simulink model "Bicycle_model"  (R2024b)
settings: Solver=FixedStepAuto  StartTime=0.0  StopTime=40  FixedStep=0.01  RelTol=1e-3
values from neighbouring files (symbols this model uses):
  a = 1.10    (= 1.1)    [Bicycle_model_parameters_formula.m]
  A = 1.80    (= 1.8)    [Bicycle_model_parameters_formula.m]
  a1f = -1e-5    (= -1e-05)    [Bicycle_model_parameters_formula.m]
  a1r = -1e-5    (= -1e-05)    [Bicycle_model_parameters_formula.m]
  a2f = 0.95    [Bicycle_model_parameters_formula.m]
  a2r = 0.95    [Bicycle_model_parameters_formula.m]
  b = L-a    (= 1.7)    [Bicycle_model_parameters_formula.m]
  Bf = 0.0813    [Bicycle_model_parameters_formula.m]
  Br = 0.0925    [Bicycle_model_parameters_formula.m]
  Cf = 1.2947    [Bicycle_model_parameters_formula.m]
  Cr = 1.2617    [Bicycle_model_parameters_formula.m]
  cz = 0    [Bicycle_model_parameters_formula.m]
  Ef = -8.3966    [Bicycle_model_parameters_formula.m]
  Er = -8.7012    [Bicycle_model_parameters_formula.m]
  g = 9.81    [Bicycle_model_parameters_formula.m]
  I = 3500    [Bicycle_model_parameters_formula.m]
  L = 2.8    [Bicycle_model_parameters_formula.m]
  m = 1650    [Bicycle_model_parameters_formula.m]
  rho = 1.225    [Bicycle_model_parameters_formula.m]
  SR = 10    [Bicycle_model_parameters_formula.m]
libraries: aerolibconvert2 x5, simulink x1
settings Model: Creator=jayku  LastModifiedBy=jayku

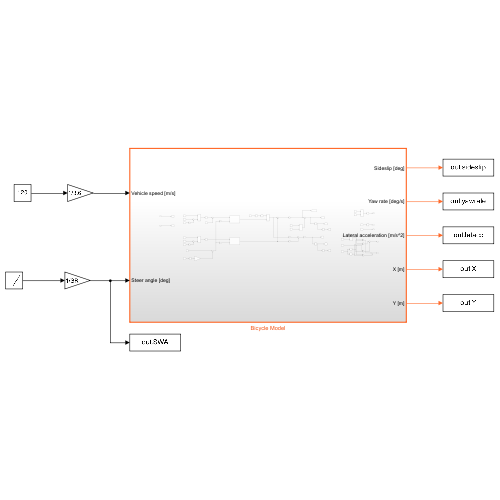
[thumbnail: Simulink's stored preview of the top-level diagram]
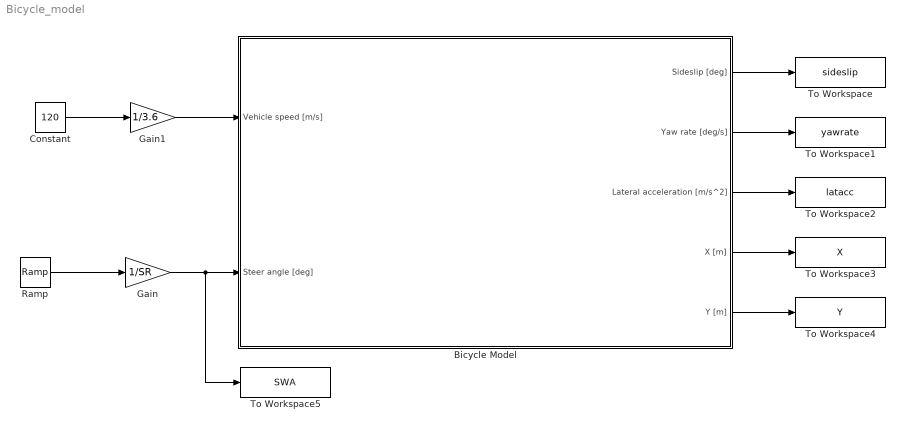
== system Bicycle_model ==
  Bicycle Model : Subsystem  TreatAsAtomicUnit=on
  Constant : Constant  Value=120
  Gain : Gain  Gain=1/SR
  Gain1 : Gain  Gain=1/3.6
  Ramp : simulink/Sources/Ramp  slope=2  start=0  InitialOutput=0
  To Workspace : ToWorkspace  VariableName=sideslip  SaveFormat=Timeseries  SampleTime=-1
  To Workspace1 : ToWorkspace  VariableName=yawrate  SaveFormat=Timeseries  SampleTime=-1
  To Workspace2 : ToWorkspace  VariableName=latacc  SaveFormat=Timeseries  SampleTime=-1
  To Workspace3 : ToWorkspace  VariableName=X  SaveFormat=Timeseries  SampleTime=-1
  To Workspace4 : ToWorkspace  VariableName=Y  SaveFormat=Timeseries  SampleTime=-1
  To Workspace5 : ToWorkspace  VariableName=SWA  SaveFormat=Timeseries  SampleTime=-1
  wires:
  Gain/1 -> To Workspace5/1, Bicycle Model/2(Steer angle [deg])
  Constant/1 -> Gain1/1
  Gain1/1 -> Bicycle Model/1(Vehicle speed [m/s])
  Ramp/1 -> Gain/1
  Bicycle Model/1(Sideslip [deg]) -> To Workspace/1
  Bicycle Model/2(Yaw rate [deg/s]) -> To Workspace1/1
  Bicycle Model/3(Lateral acceleration [m/s^2]) -> To Workspace2/1
  Bicycle Model/4(X [m]) -> To Workspace3/1
  Bicycle Model/5(Y [m]) -> To Workspace4/1

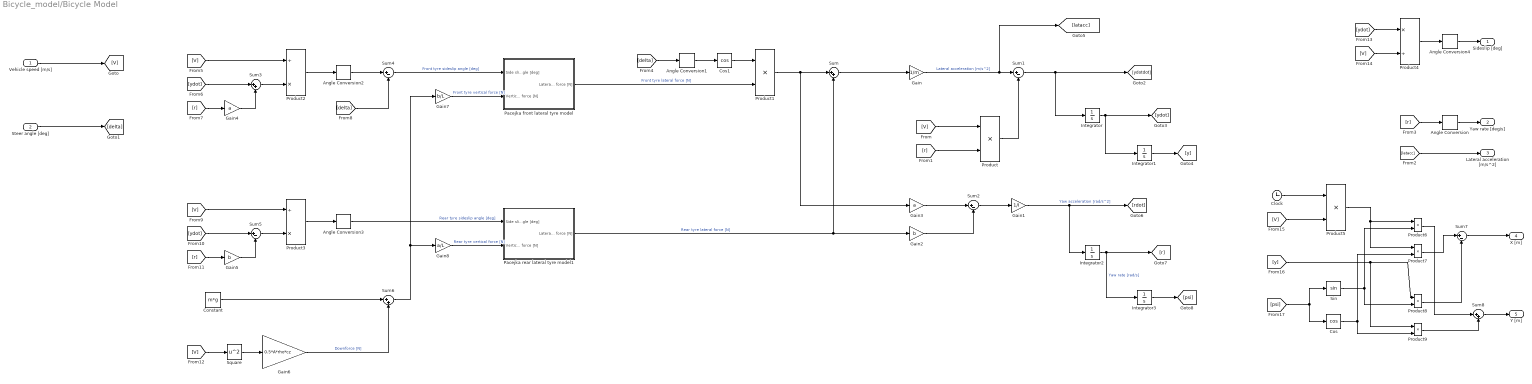
== system Bicycle_model/Bicycle Model ==
  Vehicle speed [m/s] : Inport
  Steer angle [deg] : Inport  Port=2
  Angle Conversion{,2..4} (4 alike) : aerolibconvert2/Angle Conversion  IU=rad  OU=deg
  Angle Conversion1 : aerolibconvert2/Angle Conversion  IU=deg  OU=rad
  Clock : Clock
  Constant : Constant  Value=m*g
  Cos : Trigonometry  Operator=cos
  Cos1 : Trigonometry  Operator=cos
  Gain : Gain  Gain=1/m
  Gain1 : Gain  Gain=1/I
  Gain2 : Gain  Gain=b
  Gain3 : Gain  Gain=a
  Gain4 : Gain  Gain=a
  Gain5 : Gain  Gain=b
  Gain6 : Gain  Gain=0.5*A*rho*cz
  Gain7 : Gain  Gain=b/L
  Gain8 : Gain  Gain=a/L
  Integrator{,1..3} (4 alike) : Integrator
  Pacejka front lateral tyre model : Subsystem
  Pacejka rear lateral tyre model1 : Subsystem
  Product{,1,5..9} (7 alike) : Product
  Product2 : Product  Inputs=/*
  Product3 : Product  Inputs=/*
  Product4 : Product  Inputs=*/
  Sin : Trigonometry
  Square : Math  Operator=square
  Sum{,3,6,8} (4 alike) : Sum  Inputs=|++
  Sum{1..2,4..5,7} (5 alike) : Sum  Inputs=|+-
  Sideslip [deg] : Outport
  Yaw rate [deg/s] : Outport  Port=2
  Lateral acceleration [m/s^2] : Outport  Port=3
  X [m] : Outport  Port=4
  Y [m] : Outport  Port=5
  wires:
  Vehicle speed [m/s]/1 -> [V]
  Sum/1 -> Gain/1
  Gain/1 -> [latacc], Sum1/1  "Lateral acceleration [m/s^2]"
  Product/1 -> Sum1/2
  [V] -> Product/1
  [r] -> Product/2
  Sum1/1 -> Integrator/1, [ydotdot]
  Integrator/1 -> Integrator1/1, [ydot]
  Integrator1/1 -> [y]
  [latacc] -> Lateral acceleration [m/s^2]/1
  Sum2/1 -> Gain1/1
  Gain1/1 -> Integrator2/1, [rdot]  "Yaw acceleration [rad/s^2]"
  Integrator2/1 -> [r], Integrator3/1  "Yaw rate [rad/s]"
  Integrator3/1 -> [psi]
  [r] -> Angle Conversion/1
  Angle Conversion/1 -> Yaw rate [deg/s]/1
  Gain3/1 -> Sum2/1
  Gain2/1 -> Sum2/2
  Pacejka rear lateral tyre model1/1(Lateral force [N]) -> Gain2/1, Sum/2  "Rear tyre lateral force [N]"
  Pacejka front lateral tyre model/1(Lateral force [N]) -> Product1/2  "Front tyre lateral force [N]"
  Product1/1 -> Gain3/1, Sum/1
  [delta] -> Angle Conversion1/1
  Cos1/1 -> Product1/1
  Angle Conversion1/1 -> Cos1/1
  [V] -> Product2/1
  [ydot] -> Sum3/1
  Sum3/1 -> Product2/2
  Gain4/1 -> Sum3/2
  [r] -> Gain4/1
  Product2/1 -> Angle Conversion2/1
  Angle Conversion2/1 -> Sum4/1
  [delta] -> Sum4/2
  Sum4/1 -> Pacejka front lateral tyre model/1(Side slip angle [deg])  "Front tyre sideslip angle [deg]"
  Sum5/1 -> Product3/2
  [V] -> Product3/1
  [r] -> Gain5/1
  [ydot] -> Sum5/1
  Product3/1 -> Angle Conversion3/1
  Gain5/1 -> Sum5/2
  Angle Conversion3/1 -> Pacejka rear lateral tyre model1/1(Side slip angle [deg])  "Rear tyre sideslip angle [deg]"
  Gain6/1 -> Sum6/2  "Downforce [N]"
  Constant/1 -> Sum6/1
  [V] -> Square/1
  Square/1 -> Gain6/1
  Gain8/1 -> Pacejka rear lateral tyre model1/2(Vertical force [N])  "Rear tyre vertical force [N]"
  Gain7/1 -> Pacejka front lateral tyre model/2(Vertical force [N])  "Front tyre vertical force [N]"
  Sum6/1 -> Gain7/1, Gain8/1
  Product4/1 -> Angle Conversion4/1
  Angle Conversion4/1 -> Sideslip [deg]/1
  [ydot] -> Product4/1
  [V] -> Product4/2
  Clock/1 -> Product5/1
  [V] -> Product5/2
  [psi] -> Sin/1, Cos/1
  Product5/1 -> Product7/1, Product6/1
  Sin/1 -> Product6/2, Product8/2
  Cos/1 -> Product7/2, Product9/2
  [y] -> Product9/1, Product8/1
  Product7/1 -> Sum7/1
  Product8/1 -> Sum7/2
  Product6/1 -> Sum8/1
  Product9/1 -> Sum8/2
  Sum7/1 -> X [m]/1
  Sum8/1 -> Y [m]/1
  Steer angle [deg]/1 -> [delta]

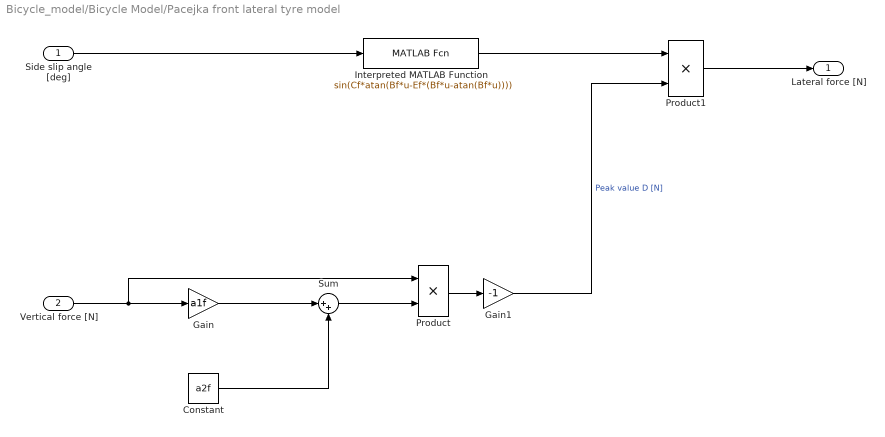
== system Bicycle_model/Bicycle Model/Pacejka front lateral tyre model ==
  Side slip angle [deg] : Inport
  Vertical force [N] : Inport  Port=2
  Constant : Constant  Value=a2f
  Gain : Gain  Gain=a1f
  Gain1 : Gain  Gain=-1
  Interpreted MATLAB Function : MATLABFcn  MATLABFcn=sin(Cf*atan(Bf*u-Ef*(Bf*u-atan(Bf*u))))
  Product : Product
  Product1 : Product
  Sum : Sum  Inputs=|++
  Lateral force [N] : Outport
  wires:
  Side slip angle [deg]/1 -> Interpreted MATLAB Function/1
  Vertical force [N]/1 -> Product/1, Gain/1
  Gain/1 -> Sum/1
  Constant/1 -> Sum/2
  Sum/1 -> Product/2
  Product/1 -> Gain1/1
  Gain1/1 -> Product1/2  "Peak value D [N]"
  Interpreted MATLAB Function/1 -> Product1/1
  Product1/1 -> Lateral force [N]/1

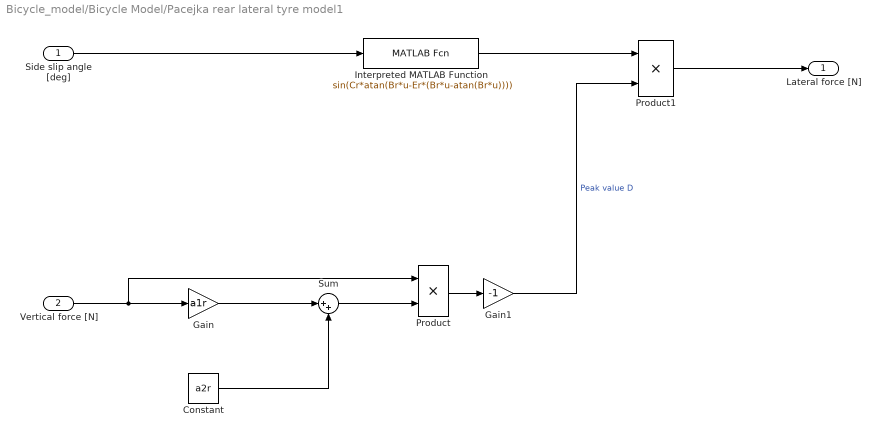
== system Bicycle_model/Bicycle Model/Pacejka rear lateral tyre model1 ==
  Side slip angle [deg] : Inport
  Vertical force [N] : Inport  Port=2
  Constant : Constant  Value=a2r
  Gain : Gain  Gain=a1r
  Gain1 : Gain  Gain=-1
  Interpreted MATLAB Function : MATLABFcn  MATLABFcn=sin(Cr*atan(Br*u-Er*(Br*u-atan(Br*u))))
  Product : Product
  Product1 : Product
  Sum : Sum  Inputs=|++
  Lateral force [N] : Outport
  wires:
  Side slip angle [deg]/1 -> Interpreted MATLAB Function/1
  Vertical force [N]/1 -> Product/1, Gain/1
  Gain/1 -> Sum/1
  Constant/1 -> Sum/2
  Sum/1 -> Product/2
  Product/1 -> Gain1/1
  Gain1/1 -> Product1/2  "Peak value D"
  Interpreted MATLAB Function/1 -> Product1/1
  Product1/1 -> Lateral force [N]/1
